simulink model "TEST_22_Aug_2020_10_26_24_be"  (R2020a)
settings: Solver=VariableStepAuto  StartTime=0.0  StopTime=30  MaxStep=0.01  RelTol=1e-3
libraries: simulink x1
settings Model: Creator=1  LastModifiedBy=1

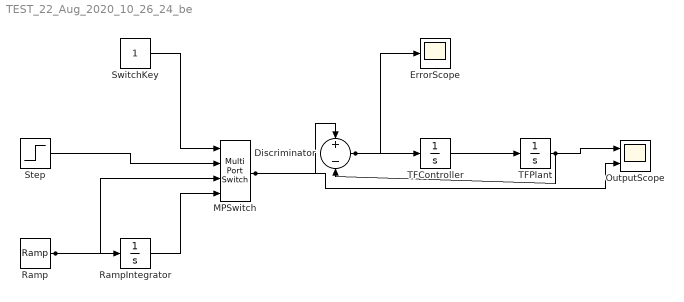
== system TEST_22_Aug_2020_10_26_24_be ==
  Discriminator : Sum  Inputs=+-
  ErrorScope : Scope
  MPSwitch : MultiPortSwitch
  OutputScope : Scope  NumInputPorts=2
  Ramp : simulink/Sources/Ramp  slope=1  start=0  InitialOutput=0
  RampIntegrator : Integrator
  Step : Step  SampleTime=0
  SwitchKey : Constant
  TFController : TransferFcn  Numerator="[0  1]"  Denominator="[1  0]"
  TFPlant : TransferFcn  Numerator="[0  1]"  Denominator="[1  0]"
  wires:
  Ramp/1 -> RampIntegrator/1, MPSwitch/3
  Step/1 -> MPSwitch/2
  RampIntegrator/1 -> MPSwitch/4
  SwitchKey/1 -> MPSwitch/1
  MPSwitch/1 -> Discriminator/1, OutputScope/2
  Discriminator/1 -> TFController/1, ErrorScope/1
  TFController/1 -> TFPlant/1
  TFPlant/1 -> OutputScope/1, Discriminator/2
